simulink model "integrated_model"  (Simulink 6.3)
settings: Solver=ode4  SolverMode=SingleTasking  StartTime=0.0  StopTime=32.0  FixedStep=0.1  RelTol=1e-3
StopFcn:
  | figure
  | subplot(332)
  | plot(re0)
  | xlabel('steps')
  | ylabel('concentration(kg/m3)')
  | subplot(334)
  | plot(re1)
  | xlabel('steps')
  | ylabel('concentration(kg/m3)')
  | subplot(335)
  | plot(re2)
  | xlabel('steps')
  | ylabel('concentration(kg/m3)')
  | subplot(336)
  | plot(re3)
  | xlabel('steps')
  | ylabel('concentration(kg/m3)')
  | subplot(337)
  | plot(re4)
  | xlabel('steps')
  | ylabel('concentration(kg/m3)')
  | subplot(338)
  | plot(re5)
  | xlabel('steps')
  | ylabel('concentration(kg/m3)')
  | subplot(339)
  | plot(re6)
  | xlabel('steps')
  | ylabel('concentration(kg/m3)')
values from neighbouring files (symbols this model uses):
  A = 8.46*1e14    (= 8.46e+14)    [all_variables_T_CO2.m]    (also in dynamic_simulink.m; ferm_integrated.m = 8.78e+14; simulink_control.m; temperatural.m = 8.78e+14)
  CO2_run = 0.13    [dynamic_simulink.m]
  flow1 = 73+7.62+flow0    (= 88.526)    [all_variables_T_CO2.m]    (also in dynamic_simulink.m = fsp1+frcy+flow0; ferm_integrated.m = str2num(get(handles.edit3,'string')); original.m = str2num(get(handles.edit3,'string')); simulink_control.m)
  flows0 = 852.21+850.02    (= 1702.23)    [all_variables_T_CO2.m]    (also in dynamic_simulink.m; simulink_control.m)
  flows1 = 852.21+850.02+850.02+752.92    (= 3305.17)    [all_variables_T_CO2.m]    (also in dynamic_simulink.m; simulink_control.m)
  flows2 = flows1+850.02    (= 4155.19)    [all_variables_T_CO2.m]    (also in dynamic_simulink.m; simulink_control.m)
  Kp = 28.779    [all_variables_T_CO2.m]    (also in dynamic_simulink.m; ferm_integrated.m; original.m; simulink_control.m)
  Kpi = 5968    [all_variables_T_CO2.m]    (also in dynamic_simulink.m; ferm_integrated.m; original.m; simulink_control.m)
  Kpp = 660.54    [all_variables_T_CO2.m]    (also in dynamic_simulink.m; ferm_integrated.m; original.m; simulink_control.m)
  Kppi = 16.658    [all_variables_T_CO2.m]    (also in dynamic_simulink.m; ferm_integrated.m; original.m; simulink_control.m)
  Kps = 9.196    [all_variables_T_CO2.m]    (also in dynamic_simulink.m; ferm_integrated.m = 9.916; original.m = 9.916; simulink_control.m)
  Kpsi = 296540    [all_variables_T_CO2.m]    (also in dynamic_simulink.m; ferm_integrated.m; original.m; simulink_control.m)
  Ks = 101.276    [all_variables_T_CO2.m]    (also in dynamic_simulink.m; ferm_integrated.m; original.m; simulink_control.m)
  Ksi = 106500    [all_variables_T_CO2.m]    (also in dynamic_simulink.m; ferm_integrated.m; original.m; simulink_control.m)
  R = 8.314    [all_variables_T_CO2.m]    (also in dynamic_simulink.m; ferm_integrated.m; simulink_control.m; temperatural.m)
  sr = 0.9886    [dynamic_simulink.m]    (also in ferm_integrated.m; original.m; temperatural.m)
  st = [10.12 1.65 218.72]    [all_variables_T_CO2.m]    (also in dynamic_simulink.m; simulink_control.m)
  Temp0 = str2num(get(handles.edit7,'string'))    [dynamic_simulink.m]    (also in simulink_control.m = str2num(get(handles.edit8,'string')))
  Temp1 = str2num(get(handles.edit9,'string'))    [dynamic_simulink.m]    (also in simulink_control.m = str2num(get(handles.edit12,'string')))
  Temp2 = str2num(get(handles.edit10,'string'))    [dynamic_simulink.m]    (also in simulink_control.m = str2num(get(handles.edit13,'string')))
  Temp3 = str2num(get(handles.edit11,'string'))    [dynamic_simulink.m]    (also in simulink_control.m = str2num(get(handles.edit14,'string')))
  Temp4 = str2num(get(handles.edit12,'string'))    [dynamic_simulink.m]    (also in simulink_control.m = str2num(get(handles.edit15,'string')))
  Temp5 = str2num(get(handles.edit13,'string'))    [dynamic_simulink.m]    (also in simulink_control.m = str2num(get(handles.edit16,'string')))
  Temp6 = str2num(get(handles.edit14,'string'))    [dynamic_simulink.m]    (also in simulink_control.m = str2num(get(handles.edit17,'string')))
  V0 = 165    [all_variables_T_CO2.m]    (also in dynamic_simulink.m; simulink_control.m)
  V1 = 600    [all_variables_T_CO2.m]    (also in dynamic_simulink.m; simulink_control.m)
  V5 = 500    [all_variables_T_CO2.m]    (also in dynamic_simulink.m; simulink_control.m)
  vmax = 0.9982    [all_variables_T_CO2.m]    (also in dynamic_simulink.m; ferm_integrated.m; original.m; simulink_control.m)
  Yps = 0.4986    [all_variables_T_CO2.m]    (also in dynamic_simulink.m; ferm_integrated.m; original.m; simulink_control.m)
  Yxs = 0.1604    [all_variables_T_CO2.m]    (also in dynamic_simulink.m; ferm_integrated.m; original.m; simulink_control.m)
settings Model: LastModifiedBy=Hyo

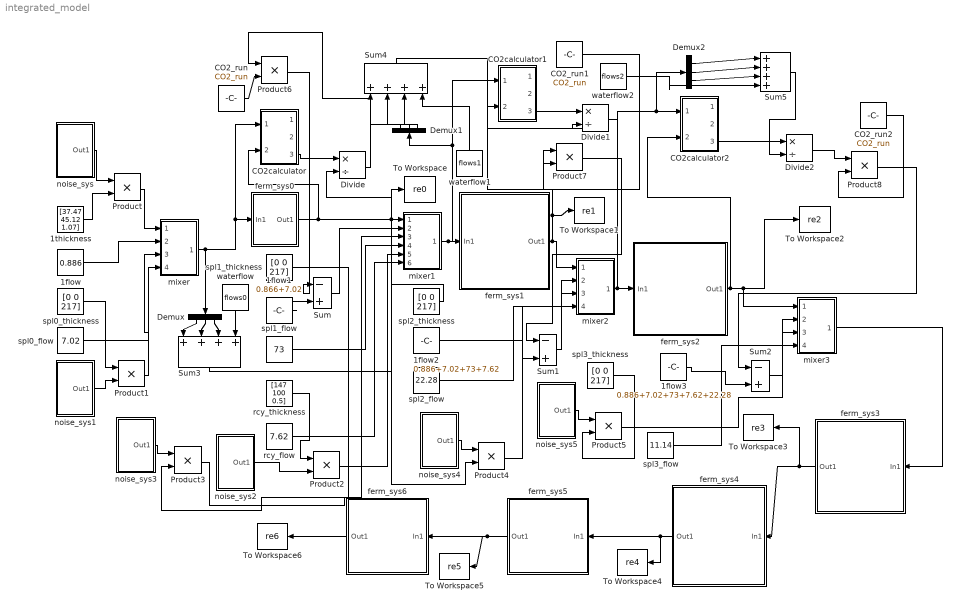
== system integrated_model ==
  1flow : Constant  Value=0.886
  1flow1 : Constant  Value=0.866+7.02
  1flow2 : Constant  Value=0.886+7.02+73+7.62
  1flow3 : Constant  Value=0.886+7.02+73+7.62+22.28  VectorParams1D=off
  1thickness : Constant  Value=[37.47 45.12 1.07]
  CO2_run : Constant  Value=CO2_run
  CO2_run1 : Constant  Value=CO2_run
  CO2_run2 : Constant  Value=CO2_run
  CO2calculator : Subsystem
  CO2calculator1 : Subsystem
  CO2calculator2 : Subsystem
  Demux : Demux  Orientation=down  Outputs=3
  Demux1 : Demux  Orientation=up  Outputs=3
  Demux2 : Demux  Outputs=3
  Divide : Product  Inputs=*/  OutScaling=2^-10
  Divide1 : Product  Inputs=*/  OutScaling=2^-10
  Divide2 : Product  Inputs=*/  OutScaling=2^-10
  Product{,1..8} (9 alike) : Product  RndMeth=Zero
  Sum : Sum  Inputs=|-+
  Sum1 : Sum  Inputs=|-+
  Sum2 : Sum  Inputs=|-+
  Sum3 : Sum  Orientation=down  Inputs=|++++
  Sum4 : Sum  Orientation=up  Inputs=|++++
  Sum5 : Sum  Inputs=|++++
  To Workspace : ToWorkspace  VariableName=re0  SampleTime=-1  SaveFormat=Array
  To Workspace1 : ToWorkspace  VariableName=re1  SampleTime=-1  SaveFormat=Array
  To Workspace2 : ToWorkspace  VariableName=re2  SampleTime=-1  SaveFormat=Array
  To Workspace3 : ToWorkspace  VariableName=re3  SampleTime=-1  SaveFormat=Array
  To Workspace4 : ToWorkspace  VariableName=re4  SampleTime=-1  SaveFormat=Array
  To Workspace5 : ToWorkspace  VariableName=re5  SampleTime=-1  SaveFormat=Array
  To Workspace6 : ToWorkspace  VariableName=re6  SampleTime=-1  SaveFormat=Array
  ferm_sys0 : Subsystem
      mask Display: image(imread('icon.jpg'));
  ferm_sys1 : Subsystem
      mask Display: image(imread('icon.jpg'));
  ferm_sys2 : Subsystem
      mask Display: image(imread('icon.jpg'));
  ferm_sys3 : Subsystem  Orientation=left
      mask Display: image(imread('icon.jpg'));
  ferm_sys4 : Subsystem  Orientation=left
      mask Display: image(imread('icon.jpg'));
  ferm_sys5 : Subsystem  Orientation=left
      mask Display: image(imread('icon.jpg'));
  ferm_sys6 : Subsystem  Orientation=left
      mask Display: image(imread('icon.jpg'));
  mixer : Subsystem
  mixer1 : Subsystem
  mixer2 : Subsystem
  mixer3 : Subsystem
  noise_sys : Subsystem
  noise_sys1 : Subsystem
  noise_sys2 : Subsystem
  noise_sys3 : Subsystem
  noise_sys4 : Subsystem
  noise_sys5 : Subsystem
  rcy_flow : Constant  Value=7.62
  rcy_thickness : Constant  Value=[147 100 0.5]
  spl0_flow : Constant  Value=7.02
  spl0_thickness : Constant  Value=[0 0 217]
  spl1_flow : Constant  Value=73
  spl1_thickness : Constant  Value=[0 0 217]
  spl2_flow : Constant  Value=22.28
  spl2_thickness : Constant  Value=[0 0 217]
  spl3_flow : Constant  Value=11.14
  spl3_thickness : Constant  Value=[0 0 217]
  waterflow : Constant  Orientation=down  Value=flows0
  waterflow1 : Constant  Orientation=up  Value=flows1
  waterflow2 : Constant  Value=flows2
  wires:
  1flow/1 -> mixer/2(In2)
  spl0_flow/1 -> mixer/4(In4)
  spl2_flow/1 -> mixer2/4(In4)
  spl3_flow/1 -> mixer3/4(In4)
  spl1_flow/1 -> mixer1/4(In4)
  rcy_flow/1 -> mixer1/6(In6)
  mixer/1(Out1) -> ferm_sys0/1(In1), CO2calculator/1(In1), Demux/1
  mixer1/1(Out1) -> ferm_sys1/1(In1), CO2calculator1/1(In1), Demux1/1
  mixer3/1(Out1) -> ferm_sys3/1(In1)
  ferm_sys6/1(Out1) -> To Workspace6/1
  ferm_sys5/1(Out1) -> ferm_sys6/1(In1), To Workspace5/1
  ferm_sys4/1(Out1) -> To Workspace4/1, ferm_sys5/1(In1)
  ferm_sys3/1(Out1) -> To Workspace3/1, ferm_sys4/1(In1)
  ferm_sys0/1(Out1) -> mixer1/1(In1), To Workspace/1, CO2calculator/2(In2)
  ferm_sys2/1(Out1) -> mixer3/1(In1), To Workspace2/1, CO2calculator2/2(In2)
  mixer2/1(Out1) -> ferm_sys2/1(In1), CO2calculator2/1(In1), Demux2/1
  ferm_sys1/1(Out1) -> mixer2/1(In1), To Workspace1/1, CO2calculator1/2(In2)
  1flow1/1 -> Sum/2
  Sum/1 -> mixer1/2(In2)
  1flow2/1 -> Sum1/2
  Sum1/1 -> mixer2/2(In2)
  1flow3/1 -> Sum2/2
  Sum2/1 -> mixer3/2(In2)
  CO2calculator/3(Out3) -> Divide/1
  Demux/1 -> Sum3/1
  Demux/2 -> Sum3/2
  Demux/3 -> Sum3/3
  Sum3/1 -> Divide/2
  CO2calculator1/3(Out3) -> Divide1/1
  Demux1/1 -> Sum4/1
  Demux1/2 -> Sum4/2
  Demux1/3 -> Sum4/3
  waterflow/1 -> Sum3/4
  waterflow1/1 -> Sum4/4
  Sum4/1 -> Divide1/2
  CO2calculator2/3(Out3) -> Divide2/1
  Demux2/1 -> Sum5/1
  Demux2/2 -> Sum5/2
  Demux2/3 -> Sum5/3
  waterflow2/1 -> Sum5/4
  Sum5/1 -> Divide2/2
  noise_sys/1(Out1) -> Product/1
  1thickness/1 -> Product/2
  Product/1 -> mixer/1(In1)
  noise_sys1/1(Out1) -> Product1/2
  spl0_thickness/1 -> Product1/1
  Product1/1 -> mixer/3(In3)
  noise_sys2/1(Out1) -> Product2/2
  rcy_thickness/1 -> Product2/1
  Product2/1 -> mixer1/5(In5)
  noise_sys3/1(Out1) -> Product3/1
  spl1_thickness/1 -> Product3/2
  Product3/1 -> mixer1/3(In3)
  noise_sys4/1(Out1) -> Product4/1
  spl2_thickness/1 -> Product4/2
  Product4/1 -> mixer2/3(In3)
  noise_sys5/1(Out1) -> Product5/1
  spl3_thickness/1 -> Product5/2
  Product5/1 -> mixer3/3(In3)
  Divide/1 -> Product6/1
  CO2_run/1 -> Product6/2
  Product6/1 -> Sum/1
  Divide1/1 -> Product7/1
  CO2_run1/1 -> Product7/2
  Product7/1 -> Sum1/1
  Divide2/1 -> Product8/1
  CO2_run2/1 -> Product8/2
  Product8/1 -> Sum2/1

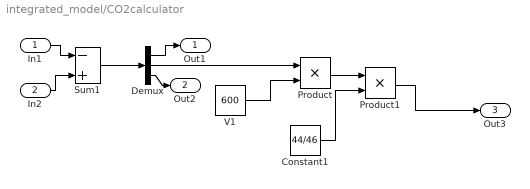
== system integrated_model/CO2calculator ==
  In1 : Inport
  In2 : Inport  Port=2
  Constant1 : Constant  Value=44/46
  Demux : Demux  Outputs=3
  Product : Product  RndMeth=Zero
  Product1 : Product  RndMeth=Zero
  Sum1 : Sum  Inputs=|-+
  V1 : Constant  Value=600
  Out1 : Outport
  Out2 : Outport  Port=2
  Out3 : Outport  Port=3
  wires:
  Sum1/1 -> Demux/1
  Demux/2 -> Product/1
  V1/1 -> Product/2
  Product/1 -> Product1/1
  Constant1/1 -> Product1/2
  Demux/1 -> Out1/1
  In1/1 -> Sum1/1
  Demux/3 -> Out2/1
  In2/1 -> Sum1/2
  Product1/1 -> Out3/1

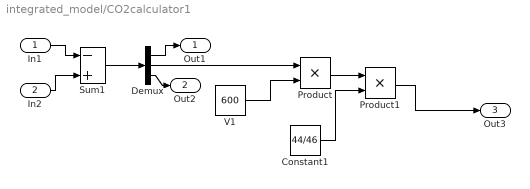
== system integrated_model/CO2calculator1 ==
  In1 : Inport
  In2 : Inport  Port=2
  Constant1 : Constant  Value=44/46
  Demux : Demux  Outputs=3
  Product : Product  RndMeth=Zero
  Product1 : Product  RndMeth=Zero
  Sum1 : Sum  Inputs=|-+
  V1 : Constant  Value=600
  Out1 : Outport
  Out2 : Outport  Port=2
  Out3 : Outport  Port=3
  wires:
  Sum1/1 -> Demux/1
  Demux/2 -> Product/1
  V1/1 -> Product/2
  Product/1 -> Product1/1
  Constant1/1 -> Product1/2
  Demux/1 -> Out1/1
  In1/1 -> Sum1/1
  Demux/3 -> Out2/1
  In2/1 -> Sum1/2
  Product1/1 -> Out3/1

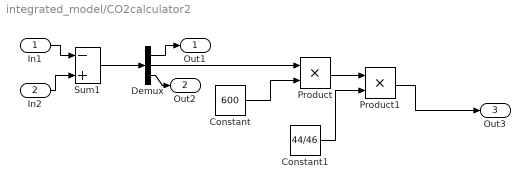
== system integrated_model/CO2calculator2 ==
  In1 : Inport
  In2 : Inport  Port=2
  Constant : Constant  Value=600
  Constant1 : Constant  Value=44/46
  Demux : Demux  Outputs=3
  Product : Product  RndMeth=Zero
  Product1 : Product  RndMeth=Zero
  Sum1 : Sum  Inputs=|-+
  Out1 : Outport
  Out2 : Outport  Port=2
  Out3 : Outport  Port=3
  wires:
  Sum1/1 -> Demux/1
  Demux/2 -> Product/1
  Constant/1 -> Product/2
  Product/1 -> Product1/1
  Constant1/1 -> Product1/2
  Demux/1 -> Out1/1
  In1/1 -> Sum1/1
  Demux/3 -> Out2/1
  In2/1 -> Sum1/2
  Product1/1 -> Out3/1

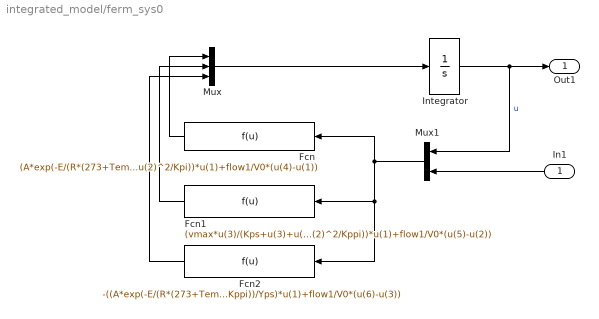
== system integrated_model/ferm_sys0 ==
  In1 : Inport  Orientation=left
  Fcn : Fcn  Orientation=left  Expr=(A*exp(-E/(R*(273+Temp0)))*u(3)/(Ks+u(3)+u(3)^2/Ksi)*Kp/(Kp+u(2)+u(2)^2/Kpi))*u(1)+flow1/V0*(u(4)-u(1))
  Fcn1 : Fcn  Orientation=left  Expr=(vmax*u(3)/(Kps+u(3)+u(3)^2/Kpsi)*Kpp/(Kpp+u(2)+u(2)^2/Kppi))*u(1)+flow1/V0*(u(5)-u(2))
  Fcn2 : Fcn  Orientation=left  Expr=-((A*exp(-E/(R*(273+Temp0)))*u(3)/(Ks+u(3)+u(3)^2/Ksi)*Kp/(Kp+u(2)+u(2)^2/Kpi))/Yxs+(vmax*u(3)/(Kps+u(3)+u(3)^2/Kpsi)*Kpp/(Kpp+u(2)+u(2)^2/Kppi))/Yps)*u(1)+flow1/V0*(u(6)-u(3))
  Integrator : Integrator  InitialCondition=st
  Mux : Mux  Inputs=3
  Mux1 : Mux  Orientation=left  Inputs=2
  Out1 : Outport
  wires:
  Integrator/1 -> Out1/1, Mux1/1  "u"
  Fcn/1 -> Mux/1
  Fcn1/1 -> Mux/2
  Fcn2/1 -> Mux/3
  Mux/1 -> Integrator/1
  In1/1 -> Mux1/2
  Mux1/1 -> Fcn/1, Fcn1/1, Fcn2/1

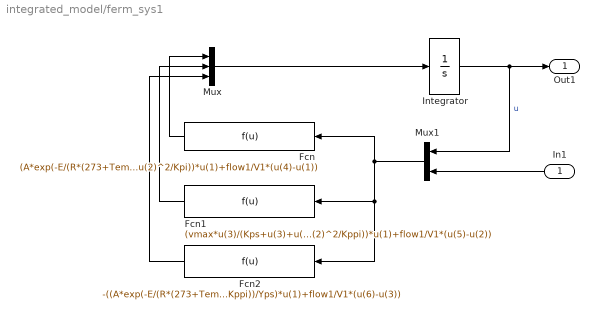
== system integrated_model/ferm_sys1 ==
  In1 : Inport  Orientation=left
  Fcn : Fcn  Orientation=left  Expr=(A*exp(-E/(R*(273+Temp1)))*u(3)/(Ks+u(3)+u(3)^2/Ksi)*Kp/(Kp+u(2)+u(2)^2/Kpi))*u(1)+flow1/V1*(u(4)-u(1))
  Fcn1 : Fcn  Orientation=left  Expr=(vmax*u(3)/(Kps+u(3)+u(3)^2/Kpsi)*Kpp/(Kpp+u(2)+u(2)^2/Kppi))*u(1)+flow1/V1*(u(5)-u(2))
  Fcn2 : Fcn  Orientation=left  Expr=-((A*exp(-E/(R*(273+Temp1)))*u(3)/(Ks+u(3)+u(3)^2/Ksi)*Kp/(Kp+u(2)+u(2)^2/Kpi))/Yxs+(vmax*u(3)/(Kps+u(3)+u(3)^2/Kpsi)*Kpp/(Kpp+u(2)+u(2)^2/Kppi))/Yps)*u(1)+flow1/V1*(u(6)-u(3))
  Integrator : Integrator  InitialCondition=st
  Mux : Mux  Inputs=3
  Mux1 : Mux  Orientation=left  Inputs=2
  Out1 : Outport
  wires:
  Integrator/1 -> Out1/1, Mux1/1  "u"
  Fcn/1 -> Mux/1
  Fcn1/1 -> Mux/2
  Fcn2/1 -> Mux/3
  Mux/1 -> Integrator/1
  In1/1 -> Mux1/2
  Mux1/1 -> Fcn/1, Fcn1/1, Fcn2/1

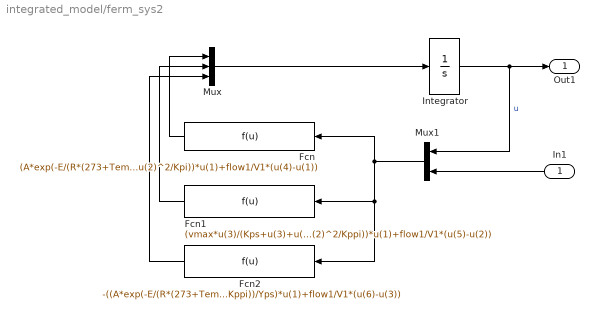
== system integrated_model/ferm_sys2 ==
  In1 : Inport  Orientation=left
  Fcn : Fcn  Orientation=left  Expr=(A*exp(-E/(R*(273+Temp2)))*u(3)/(Ks+u(3)+u(3)^2/Ksi)*Kp/(Kp+u(2)+u(2)^2/Kpi))*u(1)+flow1/V1*(u(4)-u(1))
  Fcn1 : Fcn  Orientation=left  Expr=(vmax*u(3)/(Kps+u(3)+u(3)^2/Kpsi)*Kpp/(Kpp+u(2)+u(2)^2/Kppi))*u(1)+flow1/V1*(u(5)-u(2))
  Fcn2 : Fcn  Orientation=left  Expr=-((A*exp(-E/(R*(273+Temp2)))*u(3)/(Ks+u(3)+u(3)^2/Ksi)*Kp/(Kp+u(2)+u(2)^2/Kpi))/Yxs+(vmax*u(3)/(Kps+u(3)+u(3)^2/Kpsi)*Kpp/(Kpp+u(2)+u(2)^2/Kppi))/Yps)*u(1)+flow1/V1*(u(6)-u(3))
  Integrator : Integrator  InitialCondition=st
  Mux : Mux  Inputs=3
  Mux1 : Mux  Orientation=left  Inputs=2
  Out1 : Outport
  wires:
  Integrator/1 -> Out1/1, Mux1/1  "u"
  Fcn/1 -> Mux/1
  Fcn1/1 -> Mux/2
  Fcn2/1 -> Mux/3
  Mux/1 -> Integrator/1
  In1/1 -> Mux1/2
  Mux1/1 -> Fcn/1, Fcn1/1, Fcn2/1

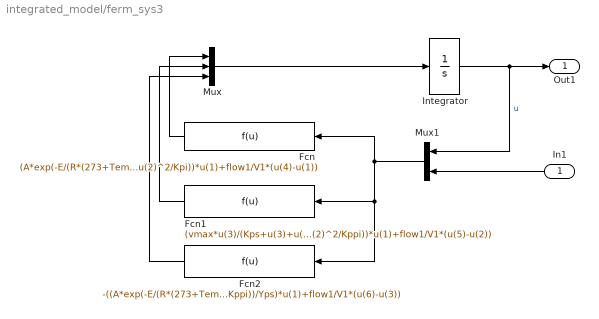
== system integrated_model/ferm_sys3 ==
  In1 : Inport  Orientation=left
  Fcn : Fcn  Orientation=left  Expr=(A*exp(-E/(R*(273+Temp3)))*u(3)/(Ks+u(3)+u(3)^2/Ksi)*Kp/(Kp+u(2)+u(2)^2/Kpi))*u(1)+flow1/V1*(u(4)-u(1))
  Fcn1 : Fcn  Orientation=left  Expr=(vmax*u(3)/(Kps+u(3)+u(3)^2/Kpsi)*Kpp/(Kpp+u(2)+u(2)^2/Kppi))*u(1)+flow1/V1*(u(5)-u(2))
  Fcn2 : Fcn  Orientation=left  Expr=-((A*exp(-E/(R*(273+Temp3)))*u(3)/(Ks+u(3)+u(3)^2/Ksi)*Kp/(Kp+u(2)+u(2)^2/Kpi))/Yxs+(vmax*u(3)/(Kps+u(3)+u(3)^2/Kpsi)*Kpp/(Kpp+u(2)+u(2)^2/Kppi))/Yps)*u(1)+flow1/V1*(u(6)-u(3))
  Integrator : Integrator  InitialCondition=st
  Mux : Mux  Inputs=3
  Mux1 : Mux  Orientation=left  Inputs=2
  Out1 : Outport
  wires:
  Integrator/1 -> Out1/1, Mux1/1  "u"
  Fcn/1 -> Mux/1
  Fcn1/1 -> Mux/2
  Fcn2/1 -> Mux/3
  Mux/1 -> Integrator/1
  In1/1 -> Mux1/2
  Mux1/1 -> Fcn/1, Fcn1/1, Fcn2/1

== system integrated_model/ferm_sys4 ==
  In1 : Inport  Orientation=left
  Fcn : Fcn  Orientation=left  Expr=(A*exp(-E/(R*(273+Temp4)))*u(3)/(Ks+u(3)+u(3)^2/Ksi)*Kp/(Kp+u(2)+u(2)^2/Kpi))*u(1)+flow1/V1*(u(4)-u(1))
  Fcn1 : Fcn  Orientation=left  Expr=(vmax*u(3)/(Kps+u(3)+u(3)^2/Kpsi)*Kpp/(Kpp+u(2)+u(2)^2/Kppi))*u(1)+flow1/V1*(u(5)-u(2))
  Fcn2 : Fcn  Orientation=left  Expr=-((A*exp(-E/(R*(273+Temp4)))*u(3)/(Ks+u(3)+u(3)^2/Ksi)*Kp/(Kp+u(2)+u(2)^2/Kpi))/Yxs+(vmax*u(3)/(Kps+u(3)+u(3)^2/Kpsi)*Kpp/(Kpp+u(2)+u(2)^2/Kppi))/Yps)*u(1)+flow1/V1*(u(6)-u(3))
  Integrator : Integrator  InitialCondition=st
  Mux : Mux  Inputs=3
  Mux1 : Mux  Orientation=left  Inputs=2
  Out1 : Outport
  wires:
  Integrator/1 -> Out1/1, Mux1/1  "u"
  Fcn/1 -> Mux/1
  Fcn1/1 -> Mux/2
  Fcn2/1 -> Mux/3
  Mux/1 -> Integrator/1
  In1/1 -> Mux1/2
  Mux1/1 -> Fcn/1, Fcn1/1, Fcn2/1

== system integrated_model/ferm_sys5 ==
  In1 : Inport  Orientation=left
  Fcn : Fcn  Orientation=left  Expr=(A*exp(-E/(R*(273+Temp5)))*u(3)/(Ks+u(3)+u(3)^2/Ksi)*Kp/(Kp+u(2)+u(2)^2/Kpi))*u(1)+flow1/V5*(u(4)-u(1))
  Fcn1 : Fcn  Orientation=left  Expr=(vmax*u(3)/(Kps+u(3)+u(3)^2/Kpsi)*Kpp/(Kpp+u(2)+u(2)^2/Kppi))*u(1)+flow1/V5*(u(5)-u(2))
  Fcn2 : Fcn  Orientation=left  Expr=-((A*exp(-E/(R*(273+Temp5)))*u(3)/(Ks+u(3)+u(3)^2/Ksi)*Kp/(Kp+u(2)+u(2)^2/Kpi))/Yxs+(vmax*u(3)/(Kps+u(3)+u(3)^2/Kpsi)*Kpp/(Kpp+u(2)+u(2)^2/Kppi))/Yps)*u(1)+flow1/V5*(u(6)-u(3))
  Integrator : Integrator  InitialCondition=st
  Mux : Mux  Inputs=3
  Mux1 : Mux  Orientation=left  Inputs=2
  Out1 : Outport
  wires:
  Integrator/1 -> Out1/1, Mux1/1  "u"
  Fcn/1 -> Mux/1
  Fcn1/1 -> Mux/2
  Fcn2/1 -> Mux/3
  Mux/1 -> Integrator/1
  In1/1 -> Mux1/2
  Mux1/1 -> Fcn/1, Fcn1/1, Fcn2/1

== system integrated_model/ferm_sys6 ==
  In1 : Inport  Orientation=left
  Fcn : Fcn  Orientation=left  Expr=(A*exp(-E/(R*(273+Temp6)))*u(3)/(Ks+u(3)+u(3)^2/Ksi)*Kp/(Kp+u(2)+u(2)^2/Kpi))*u(1)+flow1/V5*(u(4)-u(1))
  Fcn1 : Fcn  Orientation=left  Expr=(vmax*u(3)/(Kps+u(3)+u(3)^2/Kpsi)*Kpp/(Kpp+u(2)+u(2)^2/Kppi))*u(1)+flow1/V5*(u(5)-u(2))
  Fcn2 : Fcn  Orientation=left  Expr=-((A*exp(-E/(R*(273+Temp6)))*u(3)/(Ks+u(3)+u(3)^2/Ksi)*Kp/(Kp+u(2)+u(2)^2/Kpi))/Yxs+(vmax*u(3)/(Kps+u(3)+u(3)^2/Kpsi)*Kpp/(Kpp+u(2)+u(2)^2/Kppi))/Yps)*u(1)+flow1/V5*(u(6)-u(3))
  Integrator : Integrator  InitialCondition=st
  Mux : Mux  Inputs=3
  Mux1 : Mux  Orientation=left  Inputs=2
  Out1 : Outport
  wires:
  Integrator/1 -> Out1/1, Mux1/1  "u"
  Fcn/1 -> Mux/1
  Fcn1/1 -> Mux/2
  Fcn2/1 -> Mux/3
  Mux/1 -> Integrator/1
  In1/1 -> Mux1/2
  Mux1/1 -> Fcn/1, Fcn1/1, Fcn2/1

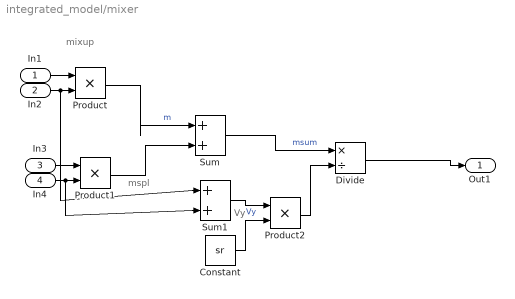
== system integrated_model/mixer ==
  note: mspl
  note: mixup
  note: Vy
  In1 : Inport
  In2 : Inport  Port=2
  In3 : Inport  Port=3
  In4 : Inport  Port=4
  Constant : Constant  Value=sr
  Divide : Product  Inputs=*/  OutScaling=2^-10
  Product : Product  RndMeth=Zero
  Product1 : Product  RndMeth=Zero
  Product2 : Product  RndMeth=Zero
  Sum : Sum  Inputs=|++
  Sum1 : Sum  Inputs=|++
  Out1 : Outport
  wires:
  In4/1 -> Product1/2, Sum1/2
  In3/1 -> Product1/1
  In2/1 -> Product/2, Sum1/1
  In1/1 -> Product/1
  Sum/1 -> Divide/1  "msum"
  Product1/1 -> Sum/2
  Product/1 -> Sum/1  "m"
  Divide/1 -> Out1/1
  Sum1/1 -> Product2/1  "Vy"
  Constant/1 -> Product2/2
  Product2/1 -> Divide/2

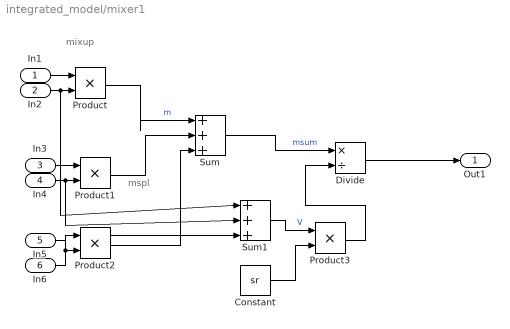
== system integrated_model/mixer1 ==
  note: mspl
  note: mixup
  In1 : Inport
  In2 : Inport  Port=2
  In3 : Inport  Port=3
  In4 : Inport  Port=4
  In5 : Inport  Port=5
  In6 : Inport  Port=6
  Constant : Constant  Value=sr
  Divide : Product  Inputs=*/  OutScaling=2^-10
  Product{,1..3} (4 alike) : Product  RndMeth=Zero
  Sum : Sum  Inputs=|+++
  Sum1 : Sum  Inputs=|+++
  Out1 : Outport
  wires:
  In4/1 -> Product1/2, Sum1/2
  In3/1 -> Product1/1
  In2/1 -> Product/2, Sum1/1
  In1/1 -> Product/1
  Sum/1 -> Divide/1  "msum"
  Product1/1 -> Sum/2
  Product/1 -> Sum/1  "m"
  In6/1 -> Product2/2, Sum1/3
  In5/1 -> Product2/1
  Product2/1 -> Sum/3
  Divide/1 -> Out1/1
  Sum1/1 -> Product3/1  "V"
  Constant/1 -> Product3/2
  Product3/1 -> Divide/2

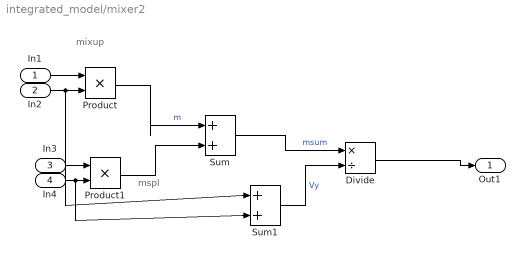
== system integrated_model/mixer2 ==
  note: mspl
  note: mixup
  In1 : Inport
  In2 : Inport  Port=2
  In3 : Inport  Port=3
  In4 : Inport  Port=4
  Divide : Product  Inputs=*/  OutScaling=2^-10
  Product : Product  RndMeth=Zero
  Product1 : Product  RndMeth=Zero
  Sum : Sum  Inputs=|++
  Sum1 : Sum  Inputs=|++
  Out1 : Outport
  wires:
  In4/1 -> Product1/2, Sum1/2
  In3/1 -> Product1/1
  In2/1 -> Product/2, Sum1/1
  In1/1 -> Product/1
  Sum1/1 -> Divide/2  "Vy"
  Sum/1 -> Divide/1  "msum"
  Product1/1 -> Sum/2
  Product/1 -> Sum/1  "m"
  Divide/1 -> Out1/1

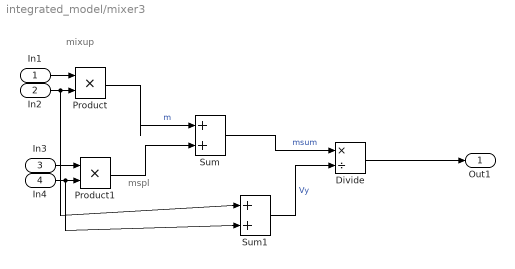
== system integrated_model/mixer3 ==
  note: mspl
  note: mixup
  In1 : Inport
  In2 : Inport  Port=2
  In3 : Inport  Port=3
  In4 : Inport  Port=4
  Divide : Product  Inputs=*/  OutScaling=2^-10
  Product : Product  RndMeth=Zero
  Product1 : Product  RndMeth=Zero
  Sum : Sum  Inputs=|++
  Sum1 : Sum  Inputs=|++
  Out1 : Outport
  wires:
  In4/1 -> Product1/2, Sum1/2
  In3/1 -> Product1/1
  In2/1 -> Product/2, Sum1/1
  In1/1 -> Product/1
  Sum1/1 -> Divide/2  "Vy"
  Sum/1 -> Divide/1  "msum"
  Product1/1 -> Sum/2
  Product/1 -> Sum/1  "m"
  Divide/1 -> Out1/1

== system integrated_model/noise_sys ==
  Constant : Constant
  Random Number : RandomNumber  Variance=0.12  SampleTime=0
  Sum : Sum  Inputs=|++
  Out1 : Outport
  wires:
  Random Number/1 -> Sum/1
  Constant/1 -> Sum/2
  Sum/1 -> Out1/1

== system integrated_model/noise_sys1 ==
  Constant : Constant
  Random Number : RandomNumber  Variance=0.12  SampleTime=0
  Sum : Sum  Inputs=|++
  Out1 : Outport
  wires:
  Random Number/1 -> Sum/1
  Constant/1 -> Sum/2
  Sum/1 -> Out1/1

== system integrated_model/noise_sys2 ==
  Constant : Constant
  Random Number : RandomNumber  Variance=0.21  SampleTime=0
  Sum : Sum  Inputs=|++
  Out1 : Outport
  wires:
  Random Number/1 -> Sum/1
  Constant/1 -> Sum/2
  Sum/1 -> Out1/1

== system integrated_model/noise_sys3 ==
  Constant : Constant
  Random Number : RandomNumber  Variance=0.12  SampleTime=0
  Sum : Sum  Inputs=|++
  Out1 : Outport
  wires:
  Random Number/1 -> Sum/1
  Constant/1 -> Sum/2
  Sum/1 -> Out1/1

== system integrated_model/noise_sys4 ==
  Constant : Constant
  Random Number : RandomNumber  Variance=0.21  SampleTime=0
  Sum : Sum  Inputs=|++
  Out1 : Outport
  wires:
  Random Number/1 -> Sum/1
  Constant/1 -> Sum/2
  Sum/1 -> Out1/1

== system integrated_model/noise_sys5 ==
  Constant : Constant
  Random Number : RandomNumber  Variance=0.21  SampleTime=0
  Sum : Sum  Inputs=|++
  Out1 : Outport
  wires:
  Random Number/1 -> Sum/1
  Constant/1 -> Sum/2
  Sum/1 -> Out1/1
